simulink model "paper"  (R2023b)
settings: Solver=FixedStepAuto  StartTime=0.0  StopTime=5  FixedStep=0.01  RelTol=1e-3
InitFcn:
  | clc;clear
  | close all
  | g = [0;2.092];
  | k1 = [-141.9203 -4.5243];
  | k2 = [-101.5134 -3.1941];
  | x0 = [0.4;-10];
settings Model: Creator=IHC  LastModifiedBy=IHC

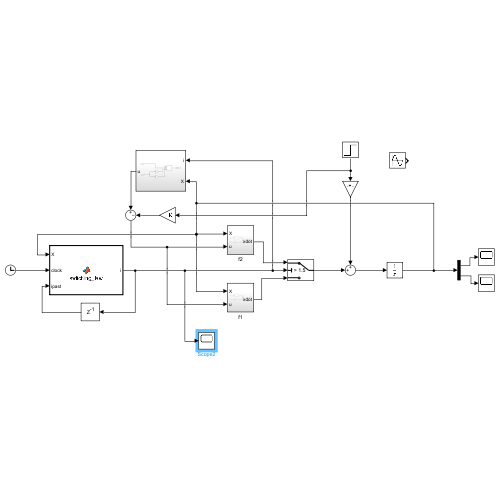
[thumbnail: Simulink's stored preview of the top-level diagram]
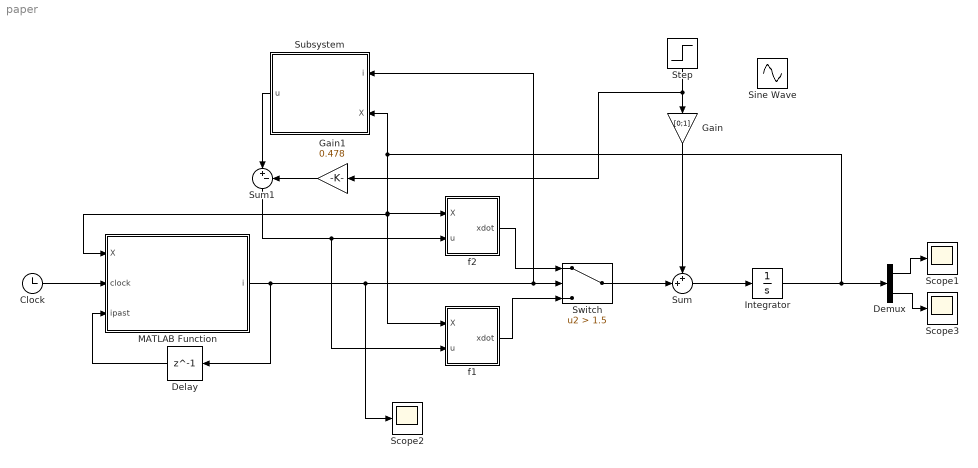
== system paper ==
  Clock : Clock
  Delay : Delay  DelayLength=1  InitialCondition=2
  Demux : Demux  Outputs=2
  Gain : Gain  Gain=[0;1]
  Gain1 : Gain  Gain=0.478
  Integrator : Integrator  InitialCondition=x0
  MATLAB Function : MATLAB Function  TreatAsAtomicUnit=on
  Scope1 : Scope
  Scope2 : Scope
  Scope3 : Scope
  Sine Wave : Sin  SampleTime=0
  Step : Step  Time=0  SampleTime=0
  Subsystem : Subsystem
  Sum : Sum  Inputs=++|
  Sum1 : Sum  Inputs=|+-
  Switch : Switch  Criteria=u2 > Threshold  Threshold=1.5  SaturateOnIntegerOverflow=off  InputSameDT=off
  f1 : Subsystem
  f2 : Subsystem
  wires:
  Clock/1 -> MATLAB Function/2(clock)
  Subsystem/1(u) -> Sum1/1
  Demux/1 -> Scope1/1
  Demux/2 -> Scope3/1
  Delay/1 -> MATLAB Function/3(ipast)
  MATLAB Function/1(i) -> Delay/1, Scope2/1, Subsystem/1(i), Switch/2
  f2/1(xdot) -> Switch/1
  f1/1(xdot) -> Switch/3
  Switch/1 -> Sum/2
  Gain/1 -> Sum/1
  Gain1/1 -> Sum1/2
  Step/1 -> Gain1/1, Gain/1
  Integrator/1 -> Demux/1, f1/1(X), MATLAB Function/1(X), f2/1(X), Subsystem/2(X)
  Sum1/1 -> f1/2(u), f2/2(u)
  Sum/1 -> Integrator/1

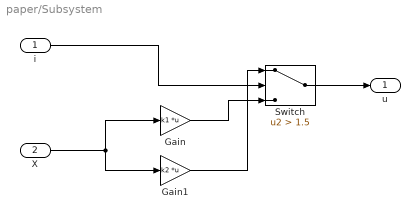
== system paper/Subsystem ==
  i : Inport
  X : Inport  Port=2
  Gain : Gain  Gain=k1  Multiplication=Matrix(K*u)
  Gain1 : Gain  Gain=k2  Multiplication=Matrix(K*u)
  Switch : Switch  Criteria=u2 > Threshold  Threshold=1.5  SaturateOnIntegerOverflow=off  InputSameDT=off
  u : Outport
  wires:
  Switch/1 -> u/1
  i/1 -> Switch/2
  X/1 -> Gain1/1, Gain/1
  Gain/1 -> Switch/3
  Gain1/1 -> Switch/1

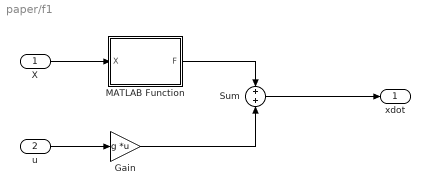
== system paper/f1 ==
  X : Inport
  u : Inport  Port=2
  Gain : Gain  Gain=g  Multiplication=Matrix(K*u)
  MATLAB Function : MATLAB Function  TreatAsAtomicUnit=on
  Sum : Sum
  xdot : Outport
  wires:
  u/1 -> Gain/1
  X/1 -> MATLAB Function/1(X)
  Gain/1 -> Sum/2
  MATLAB Function/1(F) -> Sum/1
  Sum/1 -> xdot/1

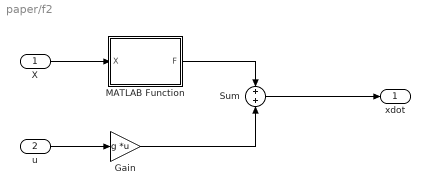
== system paper/f2 ==
  X : Inport
  u : Inport  Port=2
  Gain : Gain  Gain=g  Multiplication=Matrix(K*u)
  MATLAB Function : MATLAB Function  TreatAsAtomicUnit=on
  Sum : Sum
  xdot : Outport
  wires:
  Sum/1 -> xdot/1
  u/1 -> Gain/1
  MATLAB Function/1(F) -> Sum/1
  Gain/1 -> Sum/2
  X/1 -> MATLAB Function/1(X)

== matlab function paper/f2/MATLAB Function ==
  data: X input; F output
function F = fcn(X)
x1 = X(1);
x2 = X(2);
alpha = -7.2*10^10*(x1+0.5)*exp(-8750/(x2+350))+0.5;
beta = 1.506*10^13*(x1+0.5)*exp(-8750/(x2+350))-104.6;
f1=-2*x1+alpha;
f2 =-4.092*x2+beta;
F=[f1;f2];
end

== matlab function paper/f1/MATLAB Function ==
  data: X input; F output
function F = fcn(X)
x1 = X(1);
x2 = X(2);
alpha = -7.2*10^10*(x1+0.5)*exp(-8750/(x2+350))+0.5;
beta = 1.506*10^13*(x1+0.5)*exp(-8750/(x2+350))-104.6;
f1=-0.5*x1+alpha;
f2 =-2.592*x2+beta;
F=[f1;f2];
end

== matlab function paper/MATLAB Function ==
  data: X input; i output; clock input; ipast input
function i = switching_law(X,clock,ipast)
x1 = X(1);
x2 = X(2);
g = [0;2.092];
vx1 = zeros(1,2);
vx2 = zeros(1,2);

vx1(1,1) = [6175.531 135.679]*X;
vx1(1,2) = [135.679 4.3253]*X;
vx2(1,1) = [3590.3982 97.0491]*X;
vx2(1,2) = [97.0491 3.0536]*X;
alpha = -7.2*10^10*(x1+0.5)*exp(-8750/(x2+350))+0.5;
beta = 1.506*10^13*(x1+0.5)*exp(-8750/(x2+350))-104.6;
f1 = [-0.5*x1+alpha;-2.592*x2+beta];
f2 = [-2*x1+alpha;-4.092*x2+beta]; 
a = vx1*f1 - (1/4)*vx1*g*g'*vx1';
b = vx2*f2 - (1/4)*vx2*g*g'*vx2';

if mod(clock,0.1) == 0
    if b < a
        i = 2;
    else
        i = 1;
    end
else
    i = ipast;
end
end
